simulink model "final"  (R2020b)
settings: Solver=VariableStepAuto  StartTime=0.0  StopTime=10  RelTol=1e-3
libraries: pid_lib x3
settings Model: Creator=nevinliang  LastModifiedBy=nevinliang

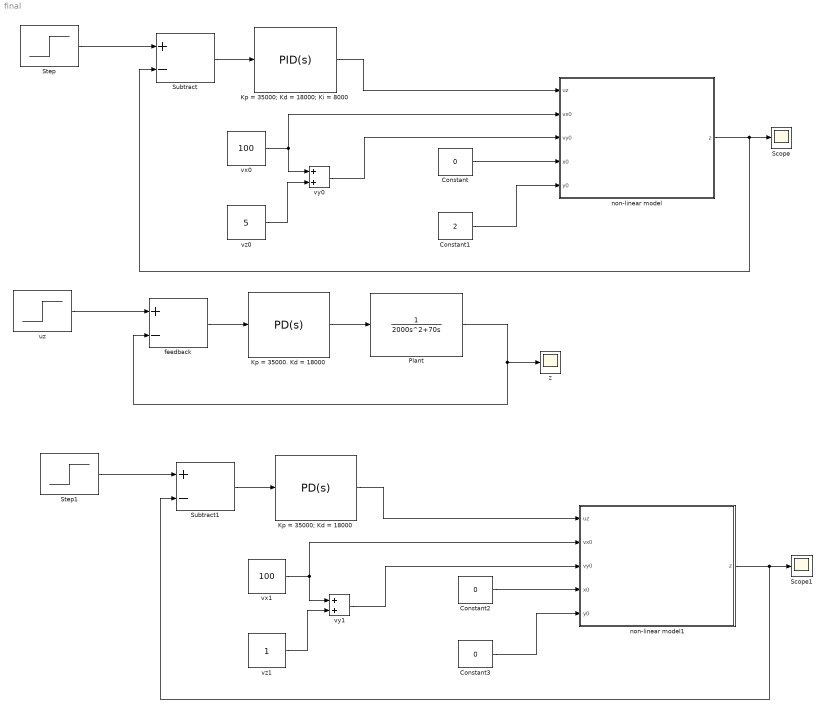
== system final ==
  Constant : Constant  Value=0
  Constant1 : Constant  Value=2
  Constant2 : Constant  Value=0
  Constant3 : Constant  Value=0
  Kp = 35000. Kd = 18000 : pid_lib/PID Controller  Controller=PD  Form=Parallel  TimeDomain=Continuous-time  UseExternalTs=off  SampleTime=-1  IntegratorMethod=Forward Euler  FilterMethod=Forward Euler  ControllerParametersSource=internal  P=35000  I=1  D=18000  UseFilter=on  N=1000  TunerSelectOption=Transfer Function Based (PID Tuner App)  InitialConditionSource=internal  InitialConditionForIntegrator=0  InitialConditionForFilter=0  DifferentiatorICPrevScaledInput=0  ExternalReset=none  TrackingMode=off  Kt=1  LimitOutput=off  SatLimitsSource=internal  UpperSaturationLimit=inf  LowerSaturationLimit=-inf  LinearizeAsGain=on  AntiWindupMode=none  Kb=1  POutMin=[]  POutMax=[]  IOutMin=[]  IOutMax=[]  DOutMin=[]  DOutMax=[]  NOutMin=[]  NOutMax=[]  SumOutMin=[]  SumOutMax=[]  SaturationOutMin=[]  SaturationOutMax=[]  PParamMin=[]  PParamMax=[]  IParamMin=[]  IParamMax=[]  DParamMin=[]  DParamMax=[]  NParamMin=[]  NParamMax=[]  KbParamMin=[]  KbParamMax=[]  KtParamMin=[]  KtParamMax=[]  KbOutMin=[]  KbOutMax=[]  KtOutMin=[]  KtOutMax=[]  IntegratorOutMin=[]  IntegratorOutMax=[]  FilterOutMin=[]  FilterOutMax=[]  SumI1OutMin=[]  SumI1OutMax=[]  SumI2OutMin=[]  SumI2OutMax=[]  SumI3OutMin=[]  SumI3OutMax=[]  SumI4OutMin=[]  SumI4OutMax=[]  SumDOutMin=[]  SumDOutMax=[]  DifferentiatorOutMin=[]  DifferentiatorOutMax=[]  FilterDiffOutCoefMin=[]  FilterDiffOutCoefMax=[]  ReciprocalOutMin=[]  ReciprocalOutMax=[]  SumDenOutMin=[]  SumDenOutMax=[]  SumNumOutMin=[]  SumNumOutMax=[]  DivideOutMin=[]  DivideOutMax=[]  UdiffTsProdOutMin=[]  UdiffTsProdOutMax=[]  NTsProdOutMin=[]  NTsProdOutMax=[]  UintegralTsProdOutMin=[]  UintegralTsProdOutMax=[]  UngainTsProdOutMin=[]  UngainTsProdOutMax=[]  IntegratorContinuousStateAttributes=''  IntegratorStateMustResolveToSignalObject=off  IntegratorRTWStateStorageClass=Auto  FilterContinuousStateAttributes=''  FilterStateMustResolveToSignalObject=off  FilterRTWStateStorageClass=Auto  ParallelPVariant=InternalParameters  IdealPVariant=Disabled  IVariant=Disabled  DVariant=InternalParameters  IntegratorVariant=Disabled  SatVariant=Disabled  AWVariant=Disabled  PCopyVariant=Disabled  TRVariant=Disabled  FdbkBlocksVariant=Forward  IdealPFdbkVariant=Disabled  SatFdbkVariant=Disabled  DerivativeFilterVariant=ContFilter  NVariant=InternalParameters  NCopyVariant=Disabled  FilterICVariant=InternalICsFilter  IntegratorICVariant=Disabled  ExternalResetVariant=Disabled  TRSumVariant=Passthrough  SumFdbkVariant=Disabled  SumVariant=Sum_PD  TsampFilterVariant=InternalTs  TsampNgainVariant=Passthrough  TsampIntegralVariant=Disabled_SignalSpec  ExternalSaturationOutDataTypeStr=Inherit: Same as second input
  Kp = 35000; Kd = 18000 : pid_lib/PID Controller  Controller=PD  Form=Parallel  TimeDomain=Continuous-time  UseExternalTs=off  SampleTime=-1  IntegratorMethod=Forward Euler  FilterMethod=Forward Euler  ControllerParametersSource=internal  P=35000  I=8000  D=18000  UseFilter=on  N=1000  TunerSelectOption=Transfer Function Based (PID Tuner App)  InitialConditionSource=internal  InitialConditionForIntegrator=0  InitialConditionForFilter=0  DifferentiatorICPrevScaledInput=0  ExternalReset=none  TrackingMode=off  Kt=1  LimitOutput=off  SatLimitsSource=internal  UpperSaturationLimit=inf  LowerSaturationLimit=-inf  LinearizeAsGain=on  AntiWindupMode=none  Kb=1  POutMin=[]  POutMax=[]  IOutMin=[]  IOutMax=[]  DOutMin=[]  DOutMax=[]  NOutMin=[]  NOutMax=[]  SumOutMin=[]  SumOutMax=[]  SaturationOutMin=[]  SaturationOutMax=[]  PParamMin=[]  PParamMax=[]  IParamMin=[]  IParamMax=[]  DParamMin=[]  DParamMax=[]  NParamMin=[]  NParamMax=[]  KbParamMin=[]  KbParamMax=[]  KtParamMin=[]  KtParamMax=[]  KbOutMin=[]  KbOutMax=[]  KtOutMin=[]  KtOutMax=[]  IntegratorOutMin=[]  IntegratorOutMax=[]  FilterOutMin=[]  FilterOutMax=[]  SumI1OutMin=[]  SumI1OutMax=[]  SumI2OutMin=[]  SumI2OutMax=[]  SumI3OutMin=[]  SumI3OutMax=[]  SumI4OutMin=[]  SumI4OutMax=[]  SumDOutMin=[]  SumDOutMax=[]  DifferentiatorOutMin=[]  DifferentiatorOutMax=[]  FilterDiffOutCoefMin=[]  FilterDiffOutCoefMax=[]  ReciprocalOutMin=[]  ReciprocalOutMax=[]  SumDenOutMin=[]  SumDenOutMax=[]  SumNumOutMin=[]  SumNumOutMax=[]  DivideOutMin=[]  DivideOutMax=[]  UdiffTsProdOutMin=[]  UdiffTsProdOutMax=[]  NTsProdOutMin=[]  NTsProdOutMax=[]  UintegralTsProdOutMin=[]  UintegralTsProdOutMax=[]  UngainTsProdOutMin=[]  UngainTsProdOutMax=[]  IntegratorContinuousStateAttributes=''  IntegratorStateMustResolveToSignalObject=off  IntegratorRTWStateStorageClass=Auto  FilterContinuousStateAttributes=''  FilterStateMustResolveToSignalObject=off  FilterRTWStateStorageClass=Auto  ParallelPVariant=InternalParameters  IdealPVariant=Disabled  IVariant=Disabled  DVariant=InternalParameters  IntegratorVariant=Disabled  SatVariant=Disabled  AWVariant=Disabled  PCopyVariant=Disabled  TRVariant=Disabled  FdbkBlocksVariant=Forward  IdealPFdbkVariant=Disabled  SatFdbkVariant=Disabled  DerivativeFilterVariant=ContFilter  NVariant=InternalParameters  NCopyVariant=Disabled  FilterICVariant=InternalICsFilter  IntegratorICVariant=Disabled  ExternalResetVariant=Disabled  TRSumVariant=Passthrough  SumFdbkVariant=Disabled  SumVariant=Sum_PD  TsampFilterVariant=InternalTs  TsampNgainVariant=Passthrough  TsampIntegralVariant=Disabled_SignalSpec  ExternalSaturationOutDataTypeStr=Inherit: Same as second input
  Kp = 35000; Kd = 18000; Ki = 8000 : pid_lib/PID Controller  Controller=PID  Form=Parallel  TimeDomain=Continuous-time  UseExternalTs=off  SampleTime=-1  IntegratorMethod=Forward Euler  FilterMethod=Forward Euler  ControllerParametersSource=internal  P=35000  I=8000  D=18000  UseFilter=on  N=1000  TunerSelectOption=Transfer Function Based (PID Tuner App)  InitialConditionSource=internal  InitialConditionForIntegrator=0  InitialConditionForFilter=0  DifferentiatorICPrevScaledInput=0  ExternalReset=none  TrackingMode=off  Kt=1  LimitOutput=off  SatLimitsSource=internal  UpperSaturationLimit=inf  LowerSaturationLimit=-inf  LinearizeAsGain=on  AntiWindupMode=none  Kb=1  POutMin=[]  POutMax=[]  IOutMin=[]  IOutMax=[]  DOutMin=[]  DOutMax=[]  NOutMin=[]  NOutMax=[]  SumOutMin=[]  SumOutMax=[]  SaturationOutMin=[]  SaturationOutMax=[]  PParamMin=[]  PParamMax=[]  IParamMin=[]  IParamMax=[]  DParamMin=[]  DParamMax=[]  NParamMin=[]  NParamMax=[]  KbParamMin=[]  KbParamMax=[]  KtParamMin=[]  KtParamMax=[]  KbOutMin=[]  KbOutMax=[]  KtOutMin=[]  KtOutMax=[]  IntegratorOutMin=[]  IntegratorOutMax=[]  FilterOutMin=[]  FilterOutMax=[]  SumI1OutMin=[]  SumI1OutMax=[]  SumI2OutMin=[]  SumI2OutMax=[]  SumI3OutMin=[]  SumI3OutMax=[]  SumI4OutMin=[]  SumI4OutMax=[]  SumDOutMin=[]  SumDOutMax=[]  DifferentiatorOutMin=[]  DifferentiatorOutMax=[]  FilterDiffOutCoefMin=[]  FilterDiffOutCoefMax=[]  ReciprocalOutMin=[]  ReciprocalOutMax=[]  SumDenOutMin=[]  SumDenOutMax=[]  SumNumOutMin=[]  SumNumOutMax=[]  DivideOutMin=[]  DivideOutMax=[]  UdiffTsProdOutMin=[]  UdiffTsProdOutMax=[]  NTsProdOutMin=[]  NTsProdOutMax=[]  UintegralTsProdOutMin=[]  UintegralTsProdOutMax=[]  UngainTsProdOutMin=[]  UngainTsProdOutMax=[]  IntegratorContinuousStateAttributes=''  IntegratorStateMustResolveToSignalObject=off  IntegratorRTWStateStorageClass=Auto  FilterContinuousStateAttributes=''  FilterStateMustResolveToSignalObject=off  FilterRTWStateStorageClass=Auto  ParallelPVariant=InternalParameters  IdealPVariant=Disabled  IVariant=InternalParameters  DVariant=InternalParameters  IntegratorVariant=Continuous  SatVariant=Disabled  AWVariant=Passthrough  PCopyVariant=Disabled  TRVariant=Disabled  FdbkBlocksVariant=Forward  IdealPFdbkVariant=Disabled  SatFdbkVariant=Disabled  DerivativeFilterVariant=ContFilter  NVariant=InternalParameters  NCopyVariant=Disabled  FilterICVariant=InternalICsFilter  IntegratorICVariant=InternalICs  ExternalResetVariant=Disabled  TRSumVariant=Passthrough  SumFdbkVariant=Disabled  SumVariant=Sum_PID  TsampFilterVariant=InternalTs  TsampNgainVariant=Passthrough  TsampIntegralVariant=Passthrough  ExternalSaturationOutDataTypeStr=Inherit: Same as second input
  Plant : TransferFcn  Denominator=[2000 70 0]
  Scope : Scope
  Scope1 : Scope
  Step : Step  Time=0  SampleTime=0
  Step1 : Step  Time=0  SampleTime=0
  Subtract : Sum  Inputs=+-
  Subtract1 : Sum  Inputs=+-
  feedback : Sum  Inputs=+-
  non-linear model : Subsystem
  non-linear model1 : Subsystem
  uz : Step  Time=0  SampleTime=0
  vx0 : Constant  Value=100
  vx1 : Constant  Value=100
  vy0 : Sum
  vy1 : Sum
  vz0 : Constant  Value=5
  vz1 : Constant
  z : Scope
  wires:
  Step/1 -> Subtract/1
  Subtract/1 -> Kp = 35000; Kd = 18000; Ki = 8000/1
  non-linear model/1(z) -> Scope/1, Subtract/2
  Kp = 35000; Kd = 18000; Ki = 8000/1 -> non-linear model/1(uz)
  vx0/1 -> vy0/1, non-linear model/2(vx0)
  uz/1 -> feedback/1
  feedback/1 -> Kp = 35000. Kd = 18000/1
  Kp = 35000. Kd = 18000/1 -> Plant/1
  Plant/1 -> feedback/2, z/1
  vy0/1 -> non-linear model/3(vy0)
  vz0/1 -> vy0/2
  Constant/1 -> non-linear model/4(x0)
  Constant1/1 -> non-linear model/5(y0)
  non-linear model1/1(z) -> Scope1/1, Subtract1/2
  Step1/1 -> Subtract1/1
  Subtract1/1 -> Kp = 35000; Kd = 18000/1
  vx1/1 -> vy1/1, non-linear model1/2(vx0)
  vy1/1 -> non-linear model1/3(vy0)
  vz1/1 -> vy1/2
  Constant3/1 -> non-linear model1/5(y0)
  Kp = 35000; Kd = 18000/1 -> non-linear model1/1(uz)
  Constant2/1 -> non-linear model1/4(x0)

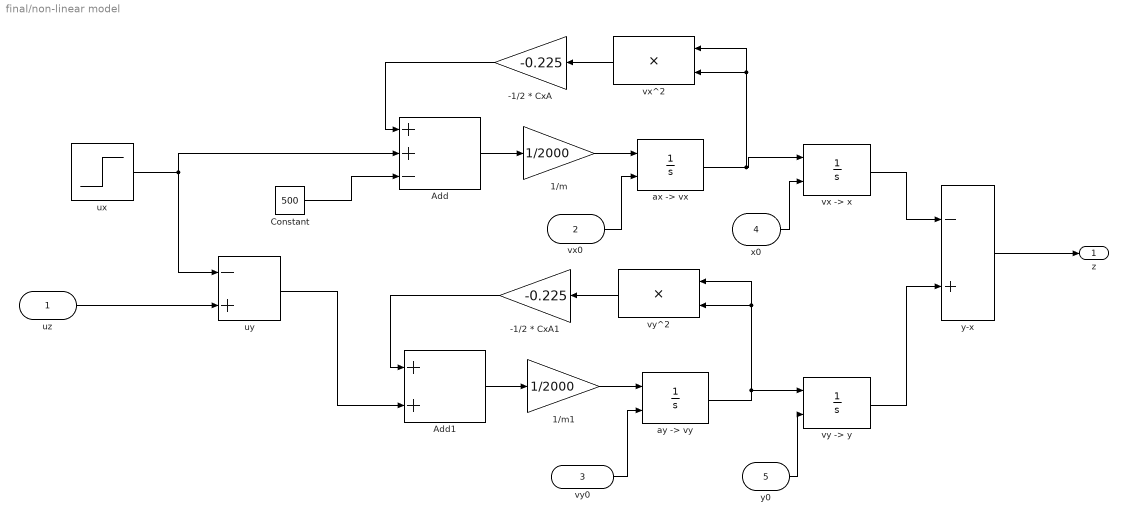
== system final/non-linear model ==
  uz : Inport
  vx0 : Inport  Port=2
  vy0 : Inport  Port=3
  x0 : Inport  Port=4
  y0 : Inport  Port=5
  -1/2 * CxA : Gain  Gain=-0.225
  -1/2 * CxA1 : Gain  Gain=-0.225
  1/m : Gain  Gain=1/2000
  1/m1 : Gain  Gain=1/2000
  Add : Sum  Inputs=++-
  Add1 : Sum
  Constant : Constant  Value=500
  "ax -> vx" : Integrator  InitialConditionSource=external
  "ay -> vy" : Integrator  InitialConditionSource=external
  ux : Step  Time=0  SampleTime=0
  uy : Sum  Inputs=-+
  "vx -> x" : Integrator  InitialConditionSource=external
  vx^2 : Product
  "vy -> y" : Integrator  InitialConditionSource=external
  vy^2 : Product
  y-x : Sum  Inputs=-+
  z : Outport
  wires:
  "ay -> vy"/1 -> vy^2/1, vy^2/2, "vy -> y"/1
  vy^2/1 -> -1/2 * CxA1/1
  "vy -> y"/1 -> y-x/2
  "ax -> vx"/1 -> vx^2/1, vx^2/2, "vx -> x"/1
  "vx -> x"/1 -> y-x/1
  -1/2 * CxA/1 -> Add/1
  Add/1 -> 1/m/1
  Add1/1 -> 1/m1/1
  ux/1 -> uy/1, Add/2
  1/m1/1 -> "ay -> vy"/1
  -1/2 * CxA1/1 -> Add1/1
  1/m/1 -> "ax -> vx"/1
  uy/1 -> Add1/2
  vx^2/1 -> -1/2 * CxA/1
  y-x/1 -> z/1
  uz/1 -> uy/2
  vx0/1 -> "ax -> vx"/2
  vy0/1 -> "ay -> vy"/2
  Constant/1 -> Add/3
  x0/1 -> "vx -> x"/2
  y0/1 -> "vy -> y"/2

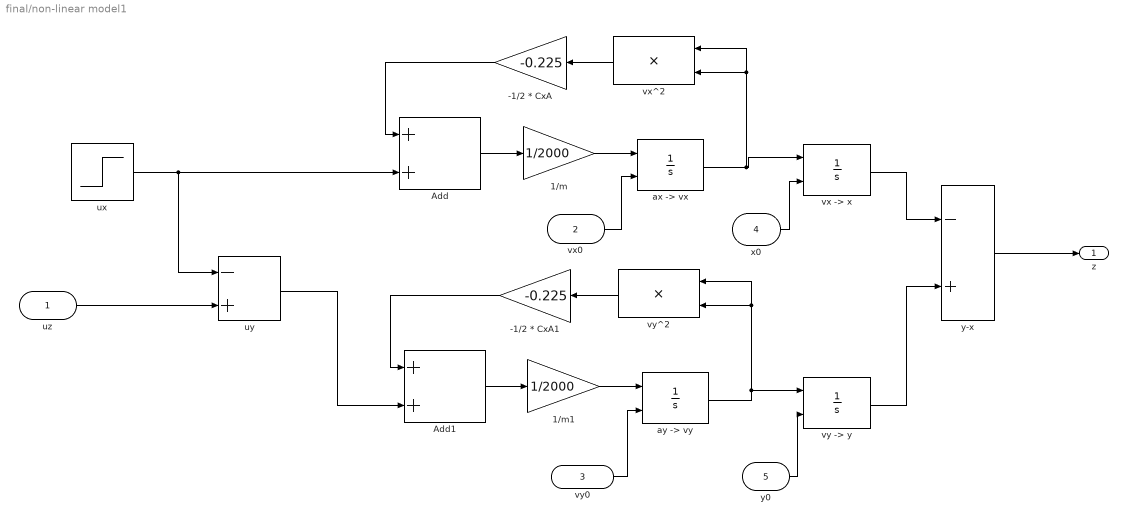
== system final/non-linear model1 ==
  uz : Inport
  vx0 : Inport  Port=2
  vy0 : Inport  Port=3
  x0 : Inport  Port=4
  y0 : Inport  Port=5
  -1/2 * CxA : Gain  Gain=-0.225
  -1/2 * CxA1 : Gain  Gain=-0.225
  1/m : Gain  Gain=1/2000
  1/m1 : Gain  Gain=1/2000
  Add : Sum
  Add1 : Sum
  "ax -> vx" : Integrator  InitialConditionSource=external
  "ay -> vy" : Integrator  InitialConditionSource=external
  ux : Step  Time=0  SampleTime=0
  uy : Sum  Inputs=-+
  "vx -> x" : Integrator  InitialConditionSource=external
  vx^2 : Product
  "vy -> y" : Integrator  InitialConditionSource=external
  vy^2 : Product
  y-x : Sum  Inputs=-+
  z : Outport
  wires:
  "ay -> vy"/1 -> vy^2/1, vy^2/2, "vy -> y"/1
  vy^2/1 -> -1/2 * CxA1/1
  "vy -> y"/1 -> y-x/2
  "ax -> vx"/1 -> vx^2/1, vx^2/2, "vx -> x"/1
  "vx -> x"/1 -> y-x/1
  -1/2 * CxA/1 -> Add/1
  Add/1 -> 1/m/1
  Add1/1 -> 1/m1/1
  ux/1 -> uy/1, Add/2
  1/m1/1 -> "ay -> vy"/1
  -1/2 * CxA1/1 -> Add1/1
  1/m/1 -> "ax -> vx"/1
  uy/1 -> Add1/2
  vx^2/1 -> -1/2 * CxA/1
  y-x/1 -> z/1
  uz/1 -> uy/2
  vx0/1 -> "ax -> vx"/2
  vy0/1 -> "ay -> vy"/2
  x0/1 -> "vx -> x"/2
  y0/1 -> "vy -> y"/2
